simulink model "NL_1DOF"  (R2019b)
settings: Solver=VariableStepAuto  StartTime=0.0  StopTime=50  RelTol=1e-3
InitFcn:
  | load("parameters.mat")
  | load("Coefficients.mat")
undefined symbols (not defined in the file): Dm, Dt, F_limit_pitch, g, Jeq, k_pitch, Mb, w_neg_0, w_neg_1, w_pos_0, w_pos_1
settings Model: Creator=peter  LastModifiedBy=peter

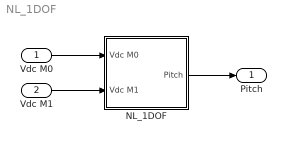
== system NL_1DOF ==
  Vdc M0 : Inport
  Vdc M1 : Inport  Port=2
  NL_1DOF : Subsystem
  Pitch : Outport
  wires:
  Vdc M0/1 -> NL_1DOF/1(Vdc M0)
  Vdc M1/1 -> NL_1DOF/2(Vdc M1)
  NL_1DOF/1(Pitch) -> Pitch/1

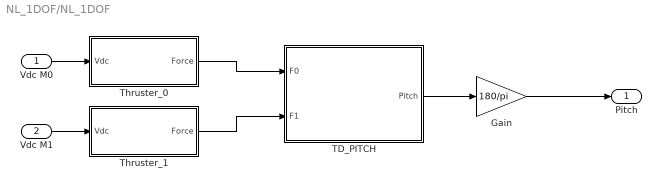
== system NL_1DOF/NL_1DOF ==
  Vdc M0 : Inport
  Vdc M1 : Inport  Port=2
  Gain : Gain  Gain=180/pi
  TD_PITCH : Subsystem
  Thruster_0 : Subsystem
  "Thruster_1 " : Subsystem
  Pitch : Outport
  wires:
  Thruster_0/1(Force) -> TD_PITCH/1(F0)
  Vdc M1/1 -> "Thruster_1 "/1(Vdc)
  TD_PITCH/1(Pitch) -> Gain/1
  "Thruster_1 "/1(Force) -> TD_PITCH/2("F1 ")
  Vdc M0/1 -> Thruster_0/1(Vdc)
  Gain/1 -> Pitch/1

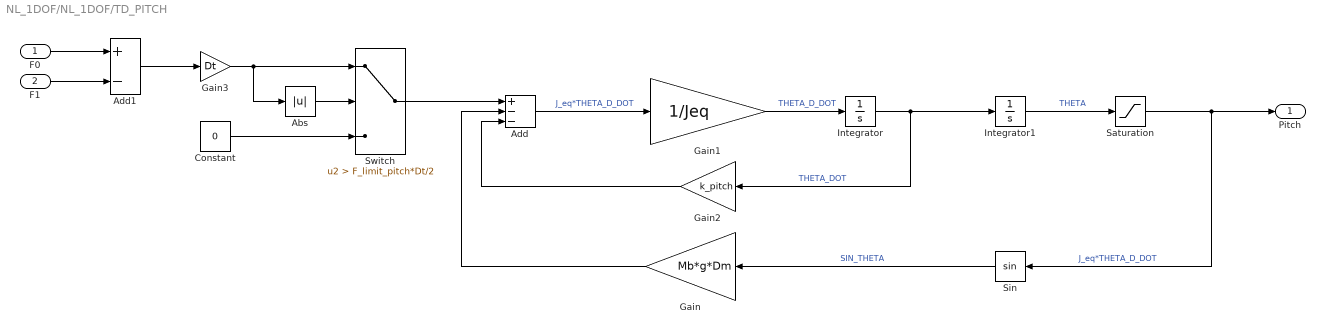
== system NL_1DOF/NL_1DOF/TD_PITCH ==
  F0 : Inport
  "F1 " : Inport  Port=2
  Abs : Abs
  Add : Sum  Inputs=+--
  Add1 : Sum  Inputs=+-
  Constant : Constant  Value=0
  Gain : Gain  Gain=Mb*g*Dm
  Gain1 : Gain  Gain=1/Jeq
  Gain2 : Gain  Gain=k_pitch
  Gain3 : Gain  Gain=Dt
  Integrator : Integrator
  Integrator1 : Integrator
  Saturation : Saturate  UpperLimit=0.93  LowerLimit=-0.93
  Sin : Trigonometry
  Switch : Switch  Criteria=u2 > Threshold  Threshold=F_limit_pitch*Dt/2
  Pitch : Outport
  wires:
  Gain2/1 -> Add/3
  Sin/1 -> Gain/1  "SIN_THETA"
  Integrator/1 -> Integrator1/1, Gain2/1  "THETA_DOT"
  Add1/1 -> Gain3/1
  Gain1/1 -> Integrator/1  "THETA_D_DOT"
  Gain/1 -> Add/2
  "F1 "/1 -> Add1/2
  Integrator1/1 -> Saturation/1  "THETA"
  F0/1 -> Add1/1
  Gain3/1 -> Abs/1, Switch/1
  Switch/1 -> Add/1
  Add/1 -> Gain1/1  "J_eq*THETA_D_DOT"
  Saturation/1 -> Pitch/1, Sin/1  "J_eq*THETA_D_DOT"
  Constant/1 -> Switch/3
  Abs/1 -> Switch/2

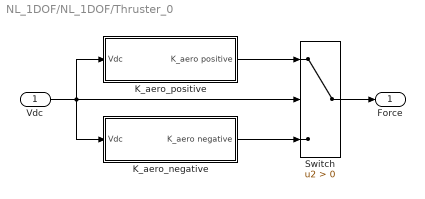
== system NL_1DOF/NL_1DOF/Thruster_0 ==
  Vdc : Inport
  K_aero_negative : Subsystem
  K_aero_positive : Subsystem
  Switch : Switch  Criteria=u2 > Threshold
  Force : Outport
  wires:
  Switch/1 -> Force/1
  K_aero_positive/1(K_aero positive) -> Switch/1
  Vdc/1 -> K_aero_positive/1(Vdc), K_aero_negative/1(Vdc), Switch/2
  K_aero_negative/1(K_aero negative) -> Switch/3

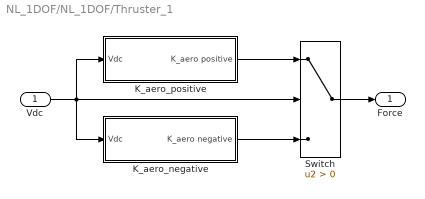
== system NL_1DOF/NL_1DOF/Thruster_1  ==
  Vdc : Inport
  K_aero_negative : Subsystem
  K_aero_positive : Subsystem
  Switch : Switch  Criteria=u2 > Threshold
  Force : Outport
  wires:
  Switch/1 -> Force/1
  K_aero_positive/1(K_aero positive) -> Switch/1
  Vdc/1 -> K_aero_negative/1(Vdc), Switch/2, K_aero_positive/1(Vdc)
  K_aero_negative/1(K_aero negative) -> Switch/3

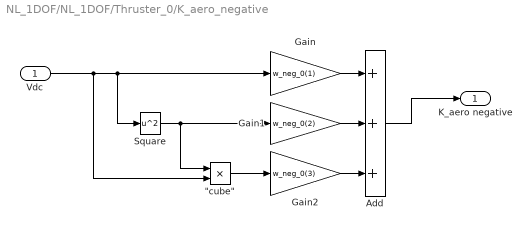
== system NL_1DOF/NL_1DOF/Thruster_0/K_aero_negative ==
  Vdc : Inport
  "\"cube\"" : Product  Inputs=**
  Add : Sum  Inputs=+++
  Gain : Gain  Gain=w_neg_0(1)
  Gain1 : Gain  Gain=w_neg_0(2)
  Gain2 : Gain  Gain=w_neg_0(3)
  Square : Math  Operator=square  SignedPower=off  SaturateOnIntegerOverflow=on
  K_aero negative : Outport
  wires:
  Vdc/1 -> "\"cube\""/2, Square/1, Gain/1
  Gain/1 -> Add/1
  Square/1 -> "\"cube\""/1, Gain1/1
  Gain1/1 -> Add/2
  Gain2/1 -> Add/3
  "\"cube\""/1 -> Gain2/1
  Add/1 -> K_aero negative/1

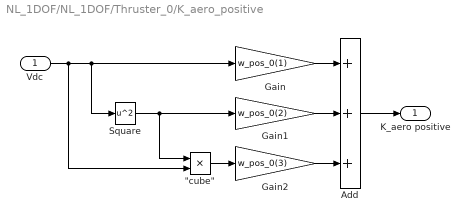
== system NL_1DOF/NL_1DOF/Thruster_0/K_aero_positive ==
  Vdc : Inport
  "\"cube\"" : Product  Inputs=**
  Add : Sum  Inputs=+++
  Gain : Gain  Gain=w_pos_0(1)
  Gain1 : Gain  Gain=w_pos_0(2)
  Gain2 : Gain  Gain=w_pos_0(3)
  Square : Math  Operator=square  SignedPower=off  SaturateOnIntegerOverflow=on
  K_aero positive : Outport
  wires:
  Vdc/1 -> Gain/1, Square/1, "\"cube\""/2
  Add/1 -> K_aero positive/1
  Gain/1 -> Add/1
  Square/1 -> "\"cube\""/1, Gain1/1
  Gain1/1 -> Add/2
  "\"cube\""/1 -> Gain2/1
  Gain2/1 -> Add/3

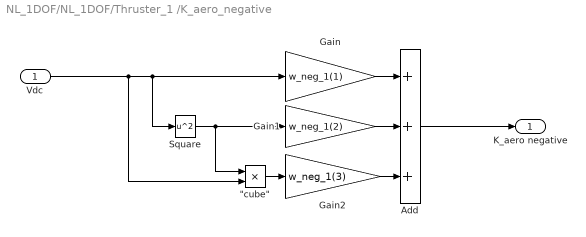
== system NL_1DOF/NL_1DOF/Thruster_1 /K_aero_negative ==
  Vdc : Inport
  "\"cube\"" : Product  Inputs=**
  Add : Sum  Inputs=+++
  Gain : Gain  Gain=w_neg_1(1)
  Gain1 : Gain  Gain=w_neg_1(2)
  Gain2 : Gain  Gain=w_neg_1(3)
  Square : Math  Operator=square  SignedPower=off  SaturateOnIntegerOverflow=on
  K_aero negative : Outport
  wires:
  Vdc/1 -> "\"cube\""/2, Square/1, Gain/1
  Gain/1 -> Add/1
  Square/1 -> "\"cube\""/1, Gain1/1
  Gain1/1 -> Add/2
  Gain2/1 -> Add/3
  "\"cube\""/1 -> Gain2/1
  Add/1 -> K_aero negative/1

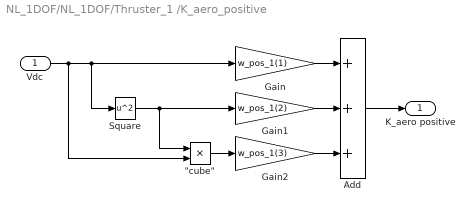
== system NL_1DOF/NL_1DOF/Thruster_1 /K_aero_positive ==
  Vdc : Inport
  "\"cube\"" : Product  Inputs=**
  Add : Sum  Inputs=+++
  Gain : Gain  Gain=w_pos_1(1)
  Gain1 : Gain  Gain=w_pos_1(2)
  Gain2 : Gain  Gain=w_pos_1(3)
  Square : Math  Operator=square  SignedPower=off  SaturateOnIntegerOverflow=on
  K_aero positive : Outport
  wires:
  Vdc/1 -> Gain/1, Square/1, "\"cube\""/2
  Add/1 -> K_aero positive/1
  Gain/1 -> Add/1
  Square/1 -> "\"cube\""/1, Gain1/1
  Gain1/1 -> Add/2
  "\"cube\""/1 -> Gain2/1
  Gain2/1 -> Add/3
